simulink model "part2_sim5"  (R2019b)
settings: Solver=FixedStepAuto  StartTime=0.0  StopTime=1500  FixedStep=0.1  RelTol=1e-3
values from neighbouring files (symbols this model uses):
  Aw = [0 0 0 -0.487387871659 0 0 0 0 0 0 -0.487387871659 0 ... (36 elements, 6x6)]    [EKFData.mat]    (also in init_observer.m = [zeros(3,3) eye(3))
  C_w = [0 0 0 0 0 0 0 0 0 1 0 0 ... (18 elements, 3x6)]    [ExtendedKalmanFilter.mat]    (also in init_wind.m = C_w.data)
  counter = 1    [init_wind.m]    (also in plotVessel.m = 2; plotVessel_thrust.m = 2)
  Cw = [0 0 0 0 0 0 0 0 0 1 0 0 ... (18 elements, 3x6)]    [EKFData.mat]    (also in init_observer.m = [zeros(3,3) eye(3)])
  D = [264860  0  0; 0  881640  0; 0  0  337740000]    [EKFData.mat]    (also in ExtendedKalmanFilter.mat; init.m = [2.6486e5, 0, 0; 0, 8.8164e5 0; 0,0, 3.3774e8])
  eta_set = [0 50 50 0 0 0 0 -50 -50 0 0 0 ... (15 elements, 5x3)]    [EKFData.mat]    (also in ExtendedKalmanFilter.mat; init_autopilot.m = [0 0 0; 50 0 0;50 -50 0; 50 -50 -pi/4; 0 -50 -pi/4; 0 0 0]; main.m = [0 0 0; 0 0 0])
  gamma_m = [0.00394784176044  0  0; 0  0.00487387871659  0; 0  0  0.00394784176044]    [EKFData.mat]    (also in ExtendedKalmanFilter.mat; init_controller.m = [omega1^2 0 0; 0 omega2^2 0; 0 0 omega3^2])
  h_step = 0.1    [init_observer.m]
  K1 = [diag([k1,k2,k3]); diag([k4 k5 k6])]    [init_observer.m]
  K2 = diag([k7,k8,k9])    [init_observer.m]
  K3 = 0.1*K4    [init_observer.m]
  K4 = 0.01*diag([1 0.3 1]).*diag(M)    [init_observer.m]
  k_lqg = lqr(A_lqg,B_lqg,Q_lqg,P_lqg)    [init_controller.m]
  K_t = eye(8)    [init_thrustalloc.m]
  Kd_matrix = [4000000  0  0; 0  5000000  0; 0  0  80000]    [EKFData.mat]    (also in ExtendedKalmanFilter.mat; init_controller.m = [4*10^(6) 0 0 ; 0 5*10^(6) 0 ; 0 0 8*10^(4)])
  Ki_matrix = [200  0  0; 0  700  0; 0  0  1000]    [EKFData.mat]    (also in ExtendedKalmanFilter.mat; init_controller.m = [2*10^(2) 0 0 ; 0 7*10^(2) 0 ; 0 0 1*10^(3)])
  Kp_matrix = [200000  0  0; 0  400000  0; 0  0  10000000]    [EKFData.mat]    (also in ExtendedKalmanFilter.mat; init_controller.m = [2*10^(5) 0 0 ; 0 4*10^(5) 0 ; 0 0 1*10^(7)])
  M_inv = [1.46677031844e-07  0  0; 0  1.2695973473e-07  9.23036390732e-11; 0  9.23036390732e-11  2.80179152408e-10]    [EKFData.mat]    (also in ExtendedKalmanFilter.mat; init_observer.m = inv(M))
  mu = 0.001    [init_wind.m]
  noise_scalar = 1    [init_observer.m]
  omega_m = [0.125663706144  0  0; 0  0.125663706144  0; 0  0  0.125663706144]    [EKFData.mat]    (also in ExtendedKalmanFilter.mat; init_controller.m = [2*zeta1*omega1 0 0; 0 2*zeta2*omega2 0;0 0 2*zeta3*omega3])
  p = 1    [EKFData.mat]    (also in ExtendedKalmanFilter.mat; init_autopilot.m)
  P0 = [0 0 0 0 0 0 0 0 0 0 0 0 ... (225 elements, 15x15)]    [EKFData.mat]    (also in ExtendedKalmanFilter.mat = [10000000 0 0 0 0 0 0 0 0 0 0 0 ... (225 elements, 15x15)]; init_observer.m = diag(ones(1,15)))
  start_time = 0    [EKFData.mat]    (also in ExtendedKalmanFilter.mat; init_autopilot.m)
  t1 = 20    [EKFData.mat]    (also in ExtendedKalmanFilter.mat; init_controller.m)
  t2 = 10    [EKFData.mat]    (also in ExtendedKalmanFilter.mat; init_controller.m = 20)
  t3 = 20    [EKFData.mat]    (also in ExtendedKalmanFilter.mat; init_controller.m)
  Tb_1 = 1000    [EKFData.mat]    (also in ExtendedKalmanFilter.mat; init_observer.m)
  thrust_loc = [l_bt1, l_bt2, l_af, l_aa, b_s, b_p]    [init_thrustalloc.m]
  thrusters =     [EKFData.mat]    (also in ExtendedKalmanFilter.mat)
  time = 0    [EKFData.mat]    (also in ExtendedKalmanFilter.mat; init_autopilot.m; plotVessel.m = Eta.time(:); plotVessel_thrust.m = Sim2.data{eta_number}.Values.time)
  vessel =     [EKFData.mat]    (also in ExtendedKalmanFilter.mat)
  x0 = [0 0 0 0 0 0 0 0 0 1 1 1 ... (15 elements, 15x1)]    [EKFData.mat]    (also in ExtendedKalmanFilter.mat = [1 1 1 1 1 1 1 1 1 1 1 1 ... (15 elements, 15x1)]; init_observer.m = zeros(15,1))
undefined symbols (not defined in the file or in its folder): Hoerner, U_gust
libraries: marine_gnc x8, simulink x7, marine_hydro x2
settings Model: Creator=jonbjor  LastModifiedBy=yngve
settings DataIOCC: ReturnWorkspaceOutputs=off
settings DebuggingCC: ArithmeticOperatorsInVariantConditions=warning
settings SFSimCC: SimUseLocalCustomCode=off  CustomCodeUndefinedFunction=UseInterfaceOnly
settings RTWCC: RTWUseLocalCustomCode=off

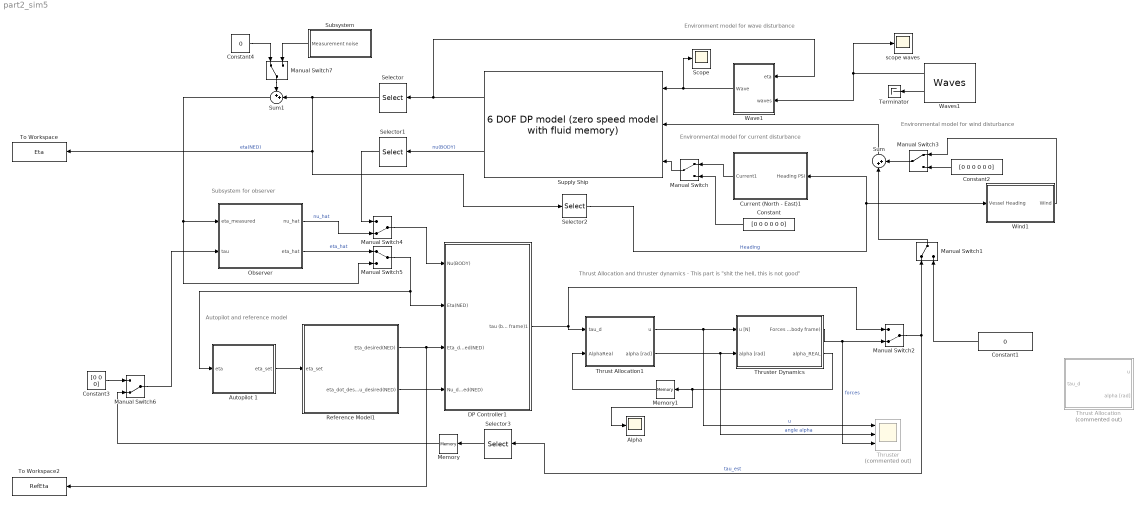
== system part2_sim5 ==
  note: Subsystem for observer
  note: Autopilot and reference model
  note: Environmental model for current disturbance
  note: Environmental model for wind disturbance
  note: Environment model for wave disturbance
  note: Thrust Allocation and thruster dynamics - This part is "shit the hell, this is not good"
  Alpha : Scope
  Autopilot 1 : Subsystem
  Constant : Constant  Value=[0 0 0 0 0 0]
  Constant1 : Constant  Value=0
  Constant2 : Constant  Value=[0 0 0 0 0 0]
  Constant3 : Constant  Value=[0 0 0]
  Constant4 : Constant  Value=0
  Current (North - East)1 : Subsystem
  DP Controller1 : Subsystem
  Manual Switch{,1,3,5,7} (5 alike) : ManualSwitch
  Manual Switch2 : ManualSwitch  CurrentSetting=0
  Manual Switch4 : ManualSwitch  CurrentSetting=0
  Manual Switch6 : ManualSwitch  CurrentSetting=0
  Memory : Memory  InheritSampleTime=on
  Memory1 : Memory  InitialCondition=[0 0 0 0 0]
  Observer : Subsystem
  Reference Model1 : Subsystem
  Scope : Scope
  Selector : Selector  InputPortWidth=6  IndexOptions=Index vector (dialog)  Indices=[1 2 6]  OutputSizes=1
  Selector1 : Selector  InputPortWidth=6  IndexOptions=Index vector (dialog)  Indices=[1 2 6]  OutputSizes=1
  Selector2 : Selector  InputPortWidth=3  IndexOptions=Index vector (dialog)  Indices=[3]  OutputSizes=1
  Selector3 : Selector  InputPortWidth=6  IndexOptions=Index vector (dialog)  Indices=[1 2 6]  OutputSizes=1
  Subsystem : Subsystem
  Sum : Sum  Inputs=|++
  Sum1 : Sum  Inputs=++|
  Supply Ship : marine_hydro/Hydro Library/6 DOF DP model  (zero speed model with fluid memory)  ABC=vesselABC  rho=1025  Axc=0.9*vessel.main.T*vessel.main.B  Ayc=0.9*vessel.main.T*vessel.main.Lpp  CX=1  CY_2D=Hoerner(vessel.main.B,vessel.main.T)  Bv=vessel.Bv  mask(6 DOF zero speed model){}
      link override "Integrator1 ": InitialCondition=nu0
      link override Integrator2: InitialCondition=eta0
      settings: SourceProductName=MSS Hydro
      mask Display:
      | image('supply.jpg');
      | color('white'); port_label('output', 1, 'eta')
      | color('white'); port_label('output', 2, 'nu')
      | color('white'); port_label('input', 1, 'tau_wave')
      | color('white'); port_label('input', 2, 'tau')
      | color('white'); port_label('input', 3, 'nu_c')
  Terminator : Terminator
  Thrust Allocation : Subsystem  Commented=on
  Thrust Allocation1 : Subsystem
  Thruster : Scope  Commented=on  NumInputPorts=3
  Thruster Dynamics : Subsystem  mask{thrusterfault=off}
      mask prompts: thrusterfault "Fault on thruster #2 and #5?"
  To Workspace : ToWorkspace  VariableName=Eta  SaveFormat=Timeseries  SampleTime=-1
  To Workspace2 : ToWorkspace  VariableName=RefEta  SaveFormat=Timeseries  SampleTime=-1
  Wave1 : Subsystem  mask{waveforces=on}
      mask prompts: waveforces "Waveforces enabled"
  Waves1 : marine_gnc/Environment/Waves/Waves  spectrum_type=Jonswap  disp_flag=on  plot_spectrum=off  plot_realization=off  hs=2.5  omega_peak=2*pi/9  psi_mean=225*pi/180  gamma=0  spread=2  depth=inf  nfreq=20  ndir=10  energylim=0.005  freq_cutoff=3  dir_cutoff=0  rand_seed=123  rand_freq=on  rand_dir=on  Zeta_a=0  Omega=0  Phase=0  Wavenum=0  Psi=0
      settings: SourceProductName=MSS GNC
  Wind1 : Subsystem
  "scope waves " : Scope
  wires:
  Selector/1 -> To Workspace/1, Selector2/1, Sum1/2  "eta(NED)"
  Observer/2(eta_hat) -> Manual Switch5/1  "eta_hat"
  Autopilot 1/1(eta_set) -> Reference Model1/1("eta_set ")
  Manual Switch1/1 -> Sum/1
  Constant/1 -> Manual Switch/2
  Manual Switch5/1 -> Autopilot 1/1(eta), DP Controller1/2("Eta(NED) ")
  Thruster Dynamics/1("Forces (body frame) ") -> Thruster/3, Manual Switch2/2  "forces"
  Supply Ship/1 -> Wave1/1(eta), Selector/1
  Manual Switch4/1 -> DP Controller1/1("Nu(BODY) ")
  Observer/1(nu_hat) -> Manual Switch4/2  "nu_hat"
  Manual Switch2/1 -> Selector3/1, Manual Switch1/1  "tau_est"
  Supply Ship/2 -> Selector1/1  "nu(BODY)"
  Selector1/1 -> Manual Switch4/1
  Constant2/1 -> Manual Switch3/2
  Manual Switch/1 -> Supply Ship/3
  Selector2/1 -> Current (North - East)1/1("Heading PSI "), Wind1/1(Vessel Heading)  "Heading"
  Manual Switch3/1 -> Sum/2
  Constant1/1 -> Manual Switch1/2
  Waves1/1 -> Wave1/2(waves), "scope waves "/1
  Wave1/1(Wave) -> Supply Ship/1, Scope/1
  Reference Model1/1(Eta_desired(NED)) -> DP Controller1/3("Eta_desired(NED) "), To Workspace2/1
  Thrust Allocation1/2(alpha [rad]) -> Thruster/2, Thruster Dynamics/2(alpha [rad])  "angle alpha"
  Thrust Allocation1/1(u) -> Thruster/1, Thruster Dynamics/1(u [N])  "u"
  Sum/1 -> Supply Ship/2
  Reference Model1/2(eta_dot_desired = nu_desired(NED)) -> DP Controller1/4(Nu_desired(NED))
  Wind1/1(Wind) -> Manual Switch3/1
  Current (North - East)1/1(Current1) -> Manual Switch/1
  Waves1/2 -> Terminator/1
  DP Controller1/1(tau (body frame)1) -> Thrust Allocation1/1(tau_d), Manual Switch2/1
  Manual Switch6/1 -> Observer/2(tau)
  Memory/1 -> Manual Switch6/2
  Constant3/1 -> Manual Switch6/1
  Sum1/1 -> Observer/1("eta_measured "), Manual Switch5/2
  Selector3/1 -> Memory/1
  Manual Switch7/1 -> Sum1/1
  Subsystem/1(Measurement noise) -> Manual Switch7/2
  Constant4/1 -> Manual Switch7/1
  Thruster Dynamics/2(alpha_REAL) -> Alpha/1, Memory1/1
  Memory1/1 -> Thrust Allocation1/2(AlphaReal)

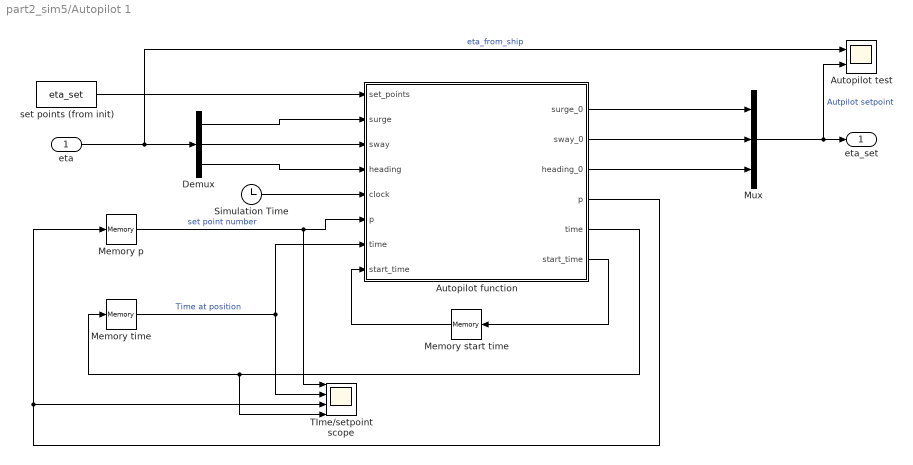
== system part2_sim5/Autopilot 1 ==
  eta : Inport
  "Autopilot function " : MATLAB Function  TreatAsAtomicUnit=on
  "Autopilot test " : Scope  NumInputPorts=2
  Demux : Demux  Outputs=3
  Memory start time : Memory  InitialCondition=start_time  InheritSampleTime=on
  Memory p : Memory  InitialCondition=p  InheritSampleTime=on
  Memory time : Memory  InitialCondition=time
  Mux : Mux  Inputs=3
  Simulation Time : Clock
  TIme/setpoint scope : Scope  NumInputPorts=4
  set points (from init) : Constant  Value=eta_set
  eta_set : Outport
  wires:
  set points (from init)/1 -> "Autopilot function "/1(set_points)
  Mux/1 -> "Autopilot test "/2, eta_set/1  "Autpilot setpoint"
  "Autopilot function "/1(surge_0) -> Mux/1
  eta/1 -> "Autopilot test "/1, Demux/1  "eta_from_ship"
  Demux/1 -> "Autopilot function "/2(surge)
  Demux/2 -> "Autopilot function "/3(sway)
  Simulation Time/1 -> "Autopilot function "/5(clock)
  Demux/3 -> "Autopilot function "/4(heading)
  "Autopilot function "/2(sway_0) -> Mux/2
  "Autopilot function "/3(heading_0) -> Mux/3
  Memory start time/1 -> "Autopilot function "/8("start_time ")
  "Autopilot function "/5(time) -> TIme/setpoint scope/4, Memory time/1
  Memory p/1 -> TIme/setpoint scope/1, "Autopilot function "/6("p ")  "set point number"
  "Autopilot function "/4(p) -> Memory p/1, TIme/setpoint scope/3
  Memory time/1 -> "Autopilot function "/7("time "), TIme/setpoint scope/2  "Time at position"
  "Autopilot function "/6(start_time) -> Memory start time/1

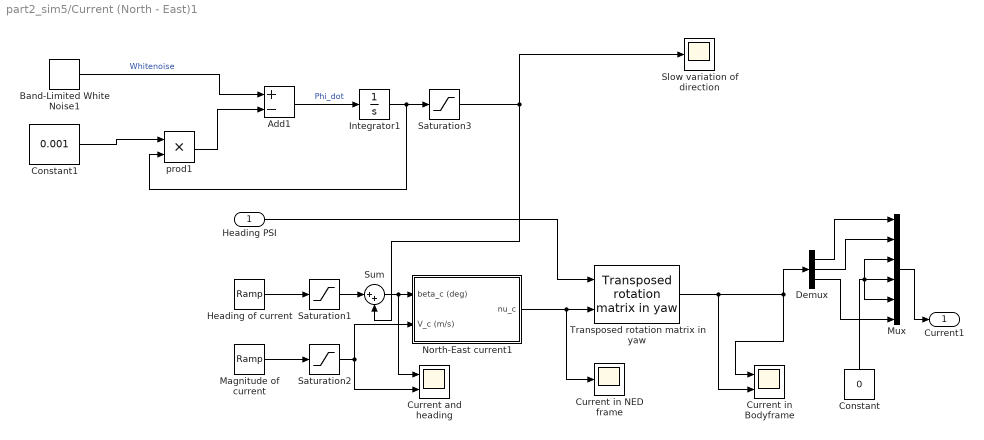
== system part2_sim5/Current (North - East)1 ==
  "Heading PSI " : Inport
  Add1 : Sum  Inputs=+-
  Band-Limited White Noise1 : simulink/Sources/Band-Limited White Noise  Cov=0.1  Ts=0.1  seed=[123456789]
  Constant : Constant  Value=0
  Constant1 : Constant  Value=0.001
  Current and heading : Scope  NumInputPorts=2
  "Current in Bodyframe " : Scope  NumInputPorts=2
  "Current in NED frame " : Scope
  Demux : Demux  Outputs=3
  "Heading of current " : simulink/Sources/Ramp  slope=0  start=0  InitialOutput=270
  Integrator1 : Integrator
  "Magnitude of current " : simulink/Sources/Ramp  slope=0  start=0  InitialOutput=0.2
  Mux : Mux  Inputs=6
  North-East current1 : Subsystem  AncestorBlock=marine_gnc/Environment/Current/North-East current
  Saturation1 : Saturate  UpperLimit=270  LowerLimit=180
  Saturation2 : Saturate  LowerLimit=0
  Saturation3 : Saturate  UpperLimit=5  LowerLimit=-5
  Slow variation of direction : Scope
  Sum : Sum  Inputs=|++
  Transposed rotation matrix in yaw : marine_gnc/Models/ Kinematics/Transposed rotation  matrix in yaw
      settings: SourceProductName=MSS GNC
  prod1 : Product  Inputs=**
  Current1 : Outport  VectorParamsAs1DForOutWhenUnconnected=off
  wires:
  Saturation2/1 -> North-East current1/2(V_c (m/s)), Current and heading/2
  "Magnitude of current "/1 -> Saturation2/1
  "Heading of current "/1 -> Saturation1/1
  Saturation1/1 -> Sum/1
  North-East current1/1(nu_c) -> Transposed rotation matrix in yaw/2, "Current in NED frame "/1
  Mux/1 -> Current1/1
  Constant/1 -> Mux/3, Mux/4, Mux/5
  Transposed rotation matrix in yaw/1 -> Demux/1, "Current in Bodyframe "/1, "Current in Bodyframe "/2
  "Heading PSI "/1 -> Transposed rotation matrix in yaw/1
  Add1/1 -> Integrator1/1  "Phi_dot"
  prod1/1 -> Add1/2
  Constant1/1 -> prod1/1
  Integrator1/1 -> Saturation3/1, prod1/2
  Band-Limited White Noise1/1 -> Add1/1  "Whitenoise"
  Saturation3/1 -> Sum/2, Slow variation of direction/1
  Sum/1 -> Current and heading/1, North-East current1/1(beta_c (deg))
  Demux/1 -> Mux/1
  Demux/2 -> Mux/2
  Demux/3 -> Mux/6

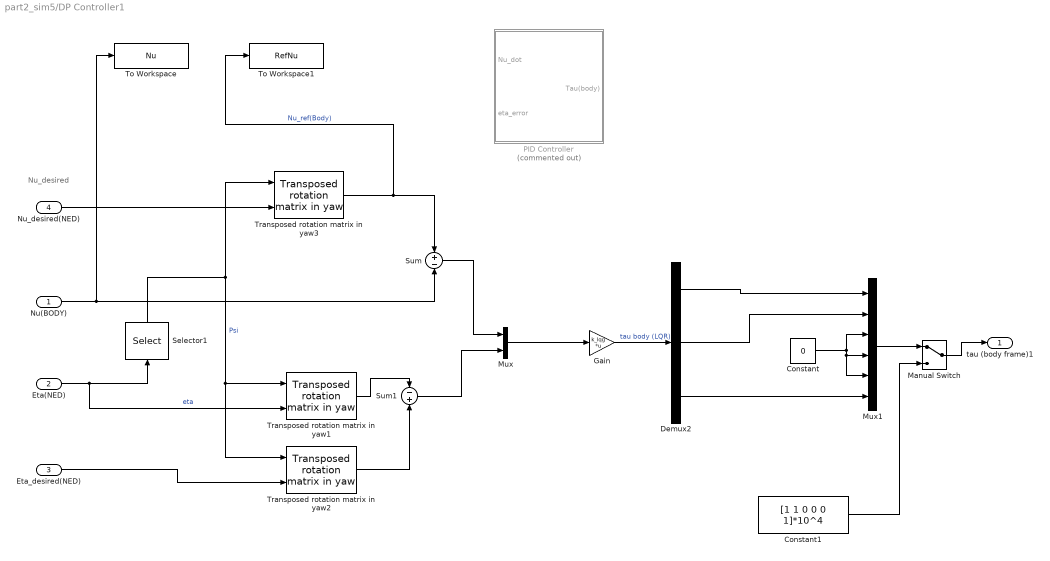
== system part2_sim5/DP Controller1 ==
  note: Nu_desired
  "Nu(BODY) " : Inport
  "Eta(NED) " : Inport  Port=2
  "Eta_desired(NED) " : Inport  Port=3
  Nu_desired(NED) : Inport  Port=4
  Constant : Constant  Value=0
  Constant1 : Constant  Value=[1 1 0 0 0 1]*10^4
  Demux2 : Demux  Outputs=3
  Gain : Gain  Gain=k_lqg  Multiplication=Matrix(K*u)
  Manual Switch : ManualSwitch
  Mux : Mux  Inputs=2
  Mux1 : Mux  Inputs=6
  "PID Controller " : Subsystem  Commented=on
  Selector1 : Selector  InputPortWidth=3  IndexOptions=Starting index (dialog)  Indices=[3]  OutputSizes=1
  Sum : Sum  Inputs=+-
  Sum1 : Sum  Inputs=-+
  To Workspace : ToWorkspace  VariableName=Nu  SaveFormat=Timeseries  SampleTime=-1
  To Workspace1 : ToWorkspace  VariableName=RefNu  SaveFormat=Timeseries  SampleTime=-1
  Transposed rotation matrix in yaw1 : marine_gnc/Models/ Kinematics/Transposed rotation  matrix in yaw
      settings: SourceProductName=MSS GNC
  Transposed rotation matrix in yaw2 : marine_gnc/Models/ Kinematics/Transposed rotation  matrix in yaw
      settings: SourceProductName=MSS GNC
  Transposed rotation matrix in yaw3 : marine_gnc/Models/ Kinematics/Transposed rotation  matrix in yaw
      settings: SourceProductName=MSS GNC
  tau (body frame)1 : Outport  VectorParamsAs1DForOutWhenUnconnected=off
  wires:
  Demux2/2 -> Mux1/2
  Selector1/1 -> Transposed rotation matrix in yaw3/1, Transposed rotation matrix in yaw2/1, Transposed rotation matrix in yaw1/1  "Psi"
  Constant/1 -> Mux1/5, Mux1/4, Mux1/3
  Demux2/1 -> Mux1/1
  "Eta(NED) "/1 -> Transposed rotation matrix in yaw1/2, Selector1/1  "eta"
  "Eta_desired(NED) "/1 -> Transposed rotation matrix in yaw2/2
  "Nu(BODY) "/1 -> To Workspace/1, Sum/2
  Nu_desired(NED)/1 -> Transposed rotation matrix in yaw3/2
  Demux2/3 -> Mux1/6
  Mux/1 -> Gain/1
  Sum/1 -> Mux/1
  Gain/1 -> Demux2/1  "tau body (LQR)"
  Transposed rotation matrix in yaw1/1 -> Sum1/1
  Sum1/1 -> Mux/2
  Transposed rotation matrix in yaw2/1 -> Sum1/2
  Transposed rotation matrix in yaw3/1 -> To Workspace1/1, Sum/1  "Nu_ref(Body)"
  Manual Switch/1 -> tau (body frame)1/1
  Mux1/1 -> Manual Switch/1
  Constant1/1 -> Manual Switch/2

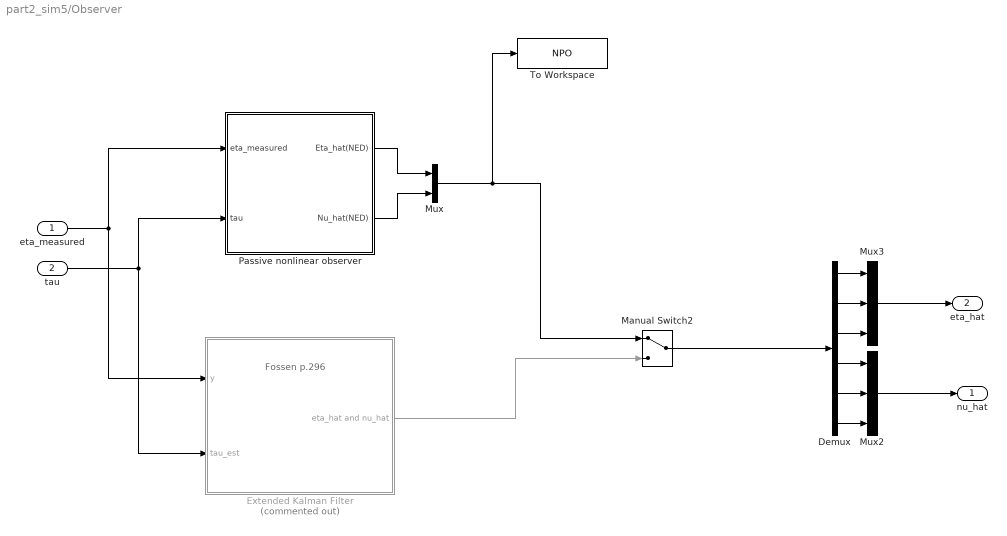
== system part2_sim5/Observer ==
  note: Fossen p.296
  "eta_measured " : Inport
  tau : Inport  Port=2  PortDimensions=[3 1]
  Demux : Demux  Outputs=6
  Extended Kalman Filter : Subsystem  Commented=on
      mask Display: image('Rudolf_Kalman.jpg'); % Use "Edit Image" on toolstrip to change.
  Manual Switch2 : ManualSwitch
  Mux : Mux  Inputs=2
  Mux2 : Mux  Inputs=3
  Mux3 : Mux  Inputs=3
  "Passive nonlinear observer " : Subsystem
  To Workspace : ToWorkspace  VariableName=NPO  SaveFormat=Timeseries  SampleTime=-1
  nu_hat : Outport
  eta_hat : Outport  Port=2
  wires:
  Extended Kalman Filter/1(eta_hat and nu_hat) -> Manual Switch2/2
  Demux/5 -> Mux2/2
  Manual Switch2/1 -> Demux/1
  Mux3/1 -> eta_hat/1
  Demux/1 -> Mux3/1
  Mux2/1 -> nu_hat/1
  Demux/3 -> Mux3/3
  Demux/6 -> Mux2/3
  Demux/4 -> Mux2/1
  Demux/2 -> Mux3/2
  tau/1 -> Extended Kalman Filter/2(tau_est), "Passive nonlinear observer "/2("tau ")
  "eta_measured "/1 -> Extended Kalman Filter/1(y), "Passive nonlinear observer "/1(eta_measured)
  "Passive nonlinear observer "/1("Eta_hat(NED) ") -> Mux/1
  "Passive nonlinear observer "/2("Nu_hat(NED) ") -> Mux/2
  Mux/1 -> To Workspace/1, Manual Switch2/1

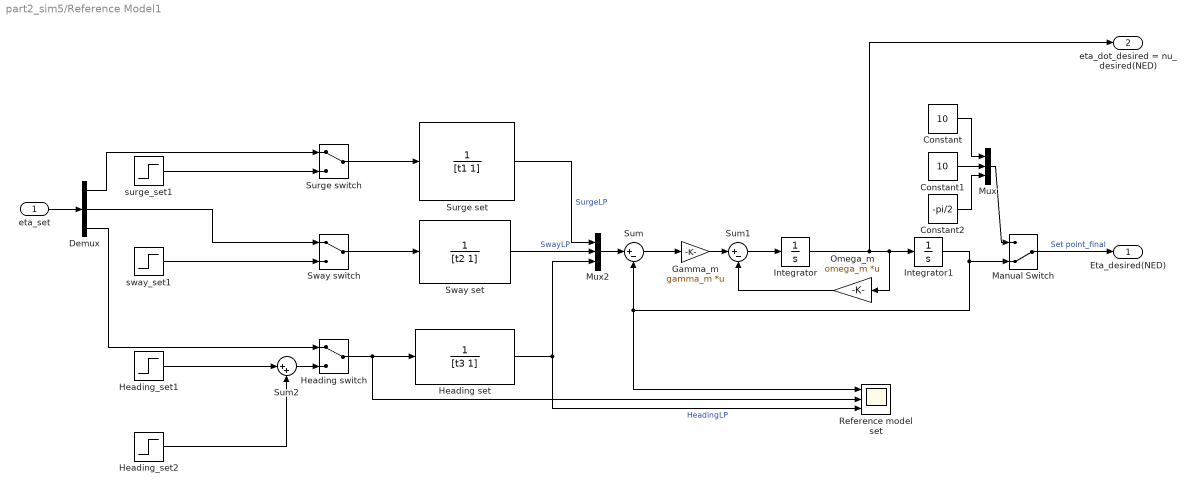
== system part2_sim5/Reference Model1 ==
  "eta_set " : Inport
  Constant : Constant  Value=10
  Constant1 : Constant  Value=10
  Constant2 : Constant  Value=-pi/2
  Demux : Demux  Outputs=3
  "Gamma_m " : Gain  Gain=gamma_m  Multiplication=Matrix(K*u)
  Heading set : TransferFcn  Denominator=[t3 1]
  "Heading switch " : ManualSwitch
  Heading_set1 : Step  Time=100  After=-pi/4  SampleTime=0
  Heading_set2 : Step  Time=800  After=pi/4  SampleTime=0
  Integrator : Integrator
  Integrator1 : Integrator
  Manual Switch : ManualSwitch  CurrentSetting=0
  Mux : Mux  Inputs=3
  Mux2 : Mux  Inputs=3
  Omega_m : Gain  Gain=omega_m  Multiplication=Matrix(K*u)
  "Reference model set " : Scope  NumInputPorts=3
  Sum : Sum  Inputs=|+-
  Sum1 : Sum  Inputs=|+-
  Sum2 : Sum  Inputs=|++
  Surge set : TransferFcn  Denominator=[t1 1]
  "Surge switch " : ManualSwitch
  Sway set : TransferFcn  Denominator=[t2 1]
  Sway switch : ManualSwitch
  "surge_set1 " : Step  Time=0  After=50  SampleTime=0
  sway_set1 : Step  Time=100  After=0  SampleTime=0
  Eta_desired(NED) : Outport  VectorParamsAs1DForOutWhenUnconnected=off
  eta_dot_desired = nu_desired(NED) : Outport  Port=2  VectorParamsAs1DForOutWhenUnconnected=off
  wires:
  Sum1/1 -> Integrator/1
  Surge set/1 -> Mux2/1  "SurgeLP"
  Sway set/1 -> Mux2/2  "SwayLP"
  Sum/1 -> "Gamma_m "/1
  Mux2/1 -> Sum/1
  Omega_m/1 -> Sum1/2
  Heading set/1 -> Mux2/3, "Reference model set "/3  "HeadingLP"
  "Gamma_m "/1 -> Sum1/1
  "Heading switch "/1 -> Heading set/1, "Reference model set "/2
  Integrator1/1 -> Manual Switch/2, "Reference model set "/1, Sum/2
  "eta_set "/1 -> Demux/1
  Demux/1 -> "Surge switch "/1
  "surge_set1 "/1 -> "Surge switch "/2
  "Surge switch "/1 -> Surge set/1
  Sway switch/1 -> Sway set/1
  sway_set1/1 -> Sway switch/2
  Demux/2 -> Sway switch/1
  Demux/3 -> "Heading switch "/1
  Heading_set1/1 -> Sum2/1
  Mux/1 -> Manual Switch/1
  Manual Switch/1 -> Eta_desired(NED)/1  "Set point_final"
  Constant/1 -> Mux/1
  Constant1/1 -> Mux/2
  Constant2/1 -> Mux/3
  Integrator/1 -> eta_dot_desired = nu_desired(NED)/1, Omega_m/1, Integrator1/1
  Sum2/1 -> "Heading switch "/2
  Heading_set2/1 -> Sum2/2

== system part2_sim5/Subsystem ==
  Band-Limited White Noise : simulink/Sources/Band-Limited White Noise  Cov=[0.01 0.01 0.01]  Ts=0.1  seed=[23341]
  Gain : Gain  Gain=noise_scalar
  Measurement noise : Outport
  wires:
  Band-Limited White Noise/1 -> Gain/1
  Gain/1 -> Measurement noise/1

== system part2_sim5/Thrust Allocation ==
  tau_d : Inport
  Constant : Constant  Value=K_t
  Constant1 : Constant  Value=thrust_loc
  MATLAB Function : MATLAB Function  TreatAsAtomicUnit=on
  Memory : Memory
  Selector : Selector  InputPortWidth=6  IndexOptions=Index vector (dialog)  Indices=[1 2 6]  OutputSizes=1
  u : Outport  VectorParamsAs1DForOutWhenUnconnected=off
  alpha [rad] : Outport  Port=2  VectorParamsAs1DForOutWhenUnconnected=off
  wires:
  tau_d/1 -> Selector/1
  MATLAB Function/1(u_thrust) -> u/1
  Constant/1 -> MATLAB Function/3(K_t)
  Constant1/1 -> MATLAB Function/2(thrust_loc)
  Selector/1 -> MATLAB Function/1(tau)
  MATLAB Function/2(alpha) -> alpha [rad]/1, Memory/1
  Memory/1 -> MATLAB Function/4(alpha_prev)

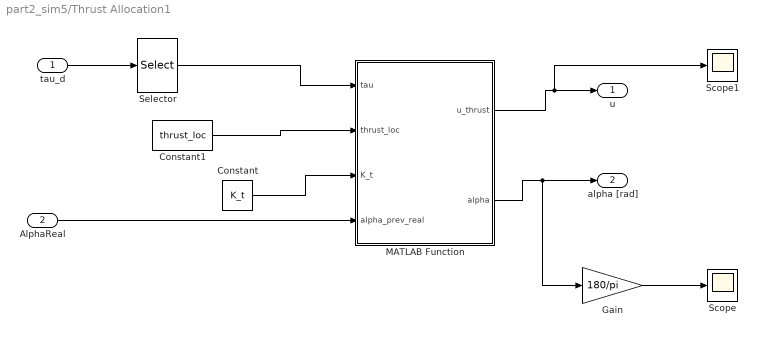
== system part2_sim5/Thrust Allocation1 ==
  tau_d : Inport
  AlphaReal : Inport  Port=2
  Constant : Constant  Value=K_t
  Constant1 : Constant  Value=thrust_loc
  Gain : Gain  Gain=180/pi
  MATLAB Function : MATLAB Function  TreatAsAtomicUnit=on
  Scope : Scope
  Scope1 : Scope
  Selector : Selector  InputPortWidth=6  IndexOptions=Index vector (dialog)  Indices=[1 2 6]  OutputSizes=1
  u : Outport  VectorParamsAs1DForOutWhenUnconnected=off
  alpha [rad] : Outport  Port=2  VectorParamsAs1DForOutWhenUnconnected=off
  wires:
  tau_d/1 -> Selector/1
  MATLAB Function/1(u_thrust) -> Scope1/1, u/1
  Selector/1 -> MATLAB Function/1(tau)
  MATLAB Function/2(alpha) -> Gain/1, alpha [rad]/1
  Gain/1 -> Scope/1
  Constant/1 -> MATLAB Function/3(K_t)
  Constant1/1 -> MATLAB Function/2(thrust_loc)
  AlphaReal/1 -> MATLAB Function/4(alpha_prev_real)

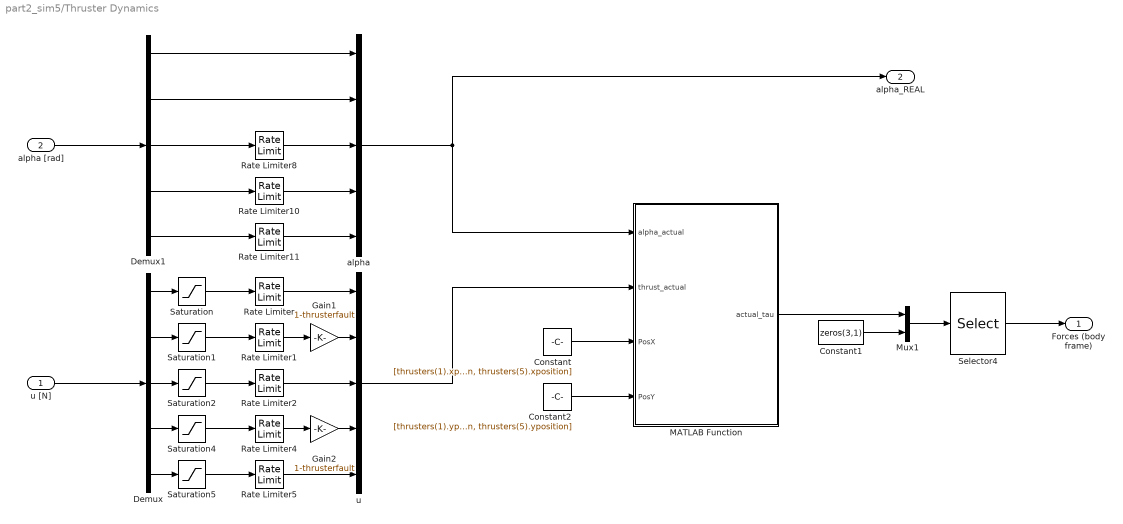
== system part2_sim5/Thruster Dynamics ==
  u [N] : Inport
  alpha [rad] : Inport  Port=2
  Constant : Constant  Value=[thrusters(1).xposition, thrusters(2).xposition, thrusters(3).xposition, thrusters(4).xposition, thrusters(5).xposition]
  Constant1 : Constant  Value=zeros(3,1)
  Constant2 : Constant  Value=[thrusters(1).yposition, thrusters(2).yposition, thrusters(3).yposition, thrusters(4).yposition, thrusters(5).yposition]
  Demux : Demux  Outputs=5
  Demux1 : Demux  Outputs=5
  Gain1 : Gain  Gain=1-thrusterfault
  Gain2 : Gain  Gain=1-thrusterfault
  MATLAB Function : MATLAB Function  TreatAsAtomicUnit=on
  Mux1 : Mux  Inputs=2
  Rate Limiter : RateLimiter  RisingSlewLimit=thrusters(1).rate  FallingSlewLimit=-thrusters(1).rate  SampleTimeMode=inherited
  Rate Limiter1 : RateLimiter  RisingSlewLimit=thrusters(2).rate  FallingSlewLimit=-thrusters(2).rate  SampleTimeMode=inherited
  Rate Limiter10 : RateLimiter  RisingSlewLimit=thrusters(4).rotationspeed  FallingSlewLimit=-thrusters(4).rotationspeed  SampleTimeMode=inherited
  Rate Limiter11 : RateLimiter  RisingSlewLimit=thrusters(5).rotationspeed  FallingSlewLimit=-thrusters(5).rotationspeed  SampleTimeMode=inherited
  Rate Limiter2 : RateLimiter  RisingSlewLimit=thrusters(3).rate  FallingSlewLimit=-thrusters(3).rate  SampleTimeMode=inherited
  Rate Limiter4 : RateLimiter  RisingSlewLimit=thrusters(4).rate  FallingSlewLimit=-thrusters(4).rate  SampleTimeMode=inherited
  Rate Limiter5 : RateLimiter  RisingSlewLimit=thrusters(5).rate  FallingSlewLimit=-thrusters(5).rate  SampleTimeMode=inherited
  Rate Limiter8 : RateLimiter  RisingSlewLimit=thrusters(3).rotationspeed  FallingSlewLimit=-thrusters(3).rotationspeed  SampleTimeMode=inherited
  Saturation : Saturate  UpperLimit=thrusters(1).thrust  LowerLimit=-thrusters(1).thrust
  Saturation1 : Saturate  UpperLimit=thrusters(2).thrust  LowerLimit=-thrusters(2).thrust
  Saturation2 : Saturate  UpperLimit=thrusters(3).thrust  LowerLimit=-thrusters(3).thrust
  Saturation4 : Saturate  UpperLimit=thrusters(4).thrust  LowerLimit=-thrusters(4).thrust
  Saturation5 : Saturate  UpperLimit=thrusters(5).thrust  LowerLimit=-thrusters(5).thrust
  Selector4 : Selector  InputPortWidth=6  IndexOptions=Index vector (dialog)  Indices=[1 2 4 5 6 3]  OutputSizes=1
  alpha : Mux  Inputs=5
  u : Mux  Inputs=5
  "Forces (body frame) " : Outport  VectorParamsAs1DForOutWhenUnconnected=off
  alpha_REAL : Outport  Port=2  VectorParamsAs1DForOutWhenUnconnected=off
  wires:
  Rate Limiter2/1 -> u/3
  Saturation/1 -> Rate Limiter/1
  Mux1/1 -> Selector4/1
  Constant1/1 -> Mux1/2
  Saturation4/1 -> Rate Limiter4/1
  Demux/2 -> Saturation1/1
  Saturation1/1 -> Rate Limiter1/1
  Demux/1 -> Saturation/1
  Demux/3 -> Saturation2/1
  Saturation2/1 -> Rate Limiter2/1
  Selector4/1 -> "Forces (body frame) "/1
  Gain1/1 -> u/2
  Rate Limiter1/1 -> Gain1/1
  Rate Limiter/1 -> u/1
  Rate Limiter4/1 -> Gain2/1
  Saturation5/1 -> Rate Limiter5/1
  Rate Limiter8/1 -> alpha/3
  u [N]/1 -> Demux/1
  alpha [rad]/1 -> Demux1/1
  Constant/1 -> MATLAB Function/3(PosX)
  Constant2/1 -> MATLAB Function/4(PosY)
  u/1 -> MATLAB Function/2(thrust_actual)
  alpha/1 -> MATLAB Function/1(alpha_actual), alpha_REAL/1
  MATLAB Function/1(actual_tau) -> Mux1/1
  Demux1/3 -> Rate Limiter8/1
  Rate Limiter10/1 -> alpha/4
  Demux1/4 -> Rate Limiter10/1
  Demux1/5 -> Rate Limiter11/1
  Rate Limiter11/1 -> alpha/5
  Demux1/2 -> alpha/2
  Demux1/1 -> alpha/1
  Gain2/1 -> u/4
  Demux/4 -> Saturation4/1
  Demux/5 -> Saturation5/1
  Rate Limiter5/1 -> u/5

== system part2_sim5/Wave1 ==
  eta : Inport
  waves : Inport  Port=2
  Gain : Gain  Gain=waveforces
  Sum : Sum
  Wave loads (U=0) : marine_hydro/Hydro Library/Wave loads (U=0)  SystemSampleTime=-1  Latency=0  AutoFrameSizeCalculation=off
      settings: SourceProductName=MSS Hydro
  Wave : Outport  VectorParamsAs1DForOutWhenUnconnected=off
  wires:
  eta/1 -> Wave loads (U=0)/1
  waves/1 -> Wave loads (U=0)/2
  Sum/1 -> Gain/1
  Wave loads (U=0)/1 -> Sum/1
  Wave loads (U=0)/2 -> Sum/2
  Gain/1 -> Wave/1

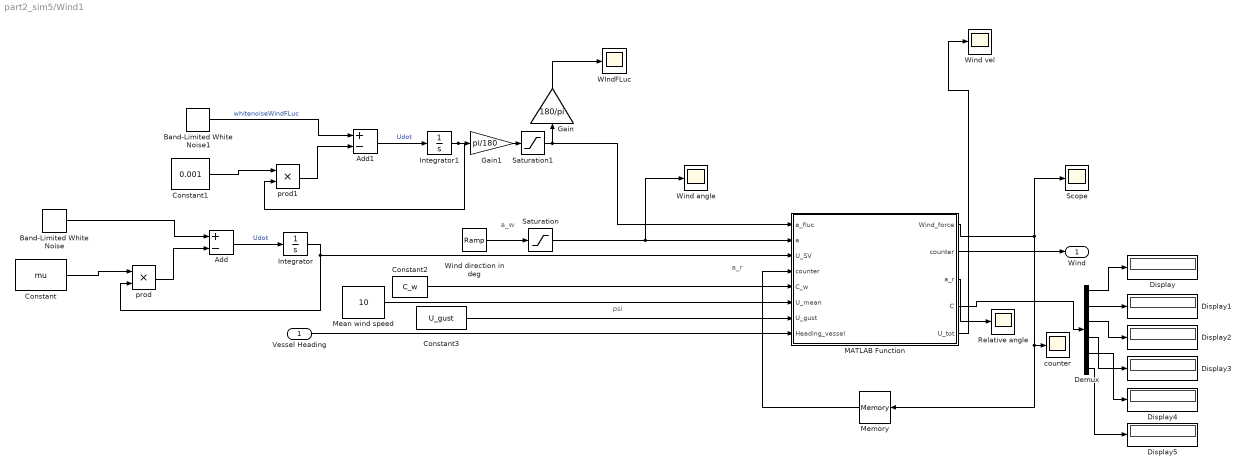
== system part2_sim5/Wind1 ==
  note: a_r
  note: psi
  note: a_w
  Vessel Heading : Inport
  Add : Sum  Inputs=+-
  Add1 : Sum  Inputs=+-
  Band-Limited White Noise : simulink/Sources/Band-Limited White Noise  Cov=w  Ts=0.1  seed=[23341]
  Band-Limited White Noise1 : simulink/Sources/Band-Limited White Noise  Cov=0.1  Ts=0.1  seed=[123456789]
  Constant : Constant  Value=mu
  Constant1 : Constant  Value=0.001
  Constant2 : Constant  Value=C_w
  Constant3 : Constant  Value=U_gust
  Demux : Demux  Outputs=6
  Display{,1..5} (6 alike) : Display
  Gain : Gain  Gain=180/pi
  Gain1 : Gain  Gain=pi/180
  Integrator : Integrator
  Integrator1 : Integrator
  MATLAB Function : MATLAB Function  TreatAsAtomicUnit=on
  Mean wind speed : Constant  Value=10
  Memory : Memory  InitialCondition=counter  InheritSampleTime=on
  "Relative angle " : Scope
  Saturation : Saturate  UpperLimit=2*pi  LowerLimit=0
  Saturation1 : Saturate  UpperLimit=5*pi/180  LowerLimit=-5*pi/180
  Scope : Scope
  "WIndFLuc " : Scope
  Wind angle : Scope
  Wind direction in deg : simulink/Sources/Ramp  slope=0  start=0  InitialOutput=pi
  "Wind vel " : Scope
  counter : Scope
  prod : Product  Inputs=**
  prod1 : Product  Inputs=**
  Wind : Outport  VectorParamsAs1DForOutWhenUnconnected=off
  wires:
  Vessel Heading/1 -> MATLAB Function/8(Heading_vessel)
  Saturation/1 -> Wind angle/1, MATLAB Function/2(a)
  Wind direction in deg/1 -> Saturation/1
  Add/1 -> Integrator/1  "Udot"
  Constant/1 -> prod/1
  Integrator/1 -> prod/2, MATLAB Function/3(U_SV)
  Band-Limited White Noise/1 -> Add/1
  prod/1 -> Add/2
  Memory/1 -> MATLAB Function/4("counter ")
  MATLAB Function/2(counter) -> Memory/1, counter/1
  Constant1/1 -> prod1/1
  Band-Limited White Noise1/1 -> Add1/1  "whitenoiseWindFLuc"
  prod1/1 -> Add1/2
  Integrator1/1 -> prod1/2, Gain1/1
  Add1/1 -> Integrator1/1  "Udot"
  MATLAB Function/1(Wind_force) -> Wind/1, Scope/1
  Constant2/1 -> MATLAB Function/5(C_w)
  Mean wind speed/1 -> MATLAB Function/6(U_mean)
  Constant3/1 -> MATLAB Function/7(U_gust)
  MATLAB Function/3(a_r) -> "Relative angle "/1
  Demux/1 -> Display/1
  Demux/2 -> Display1/1
  Demux/3 -> Display2/1
  Demux/4 -> Display3/1
  Demux/5 -> Display4/1
  Demux/6 -> Display5/1
  MATLAB Function/4(C) -> Demux/1
  MATLAB Function/5(U_tot) -> "Wind vel "/1
  Gain/1 -> "WIndFLuc "/1
  Saturation1/1 -> MATLAB Function/1(a_fluc), Gain/1
  Gain1/1 -> Saturation1/1

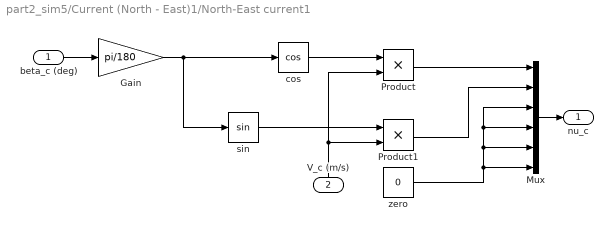
== system part2_sim5/Current (North - East)1/North-East current1 ==
  beta_c (deg) : Inport
  V_c (m/s) : Inport  Port=2
  Gain : Gain  Gain=pi/180
  Mux : Mux  Inputs=6
  Product : Product  RndMeth=Zero
  Product1 : Product  RndMeth=Zero
  cos : Trigonometry  Operator=cos
  sin : Trigonometry
  zero : Constant  Value=0
  nu_c : Outport
  wires:
  Mux/1 -> nu_c/1
  beta_c (deg)/1 -> Gain/1
  zero/1 -> Mux/6, Mux/5, Mux/4, Mux/3
  Product1/1 -> Mux/2
  Product/1 -> Mux/1
  sin/1 -> Product1/1
  V_c (m/s)/1 -> Product1/2, Product/2
  cos/1 -> Product/1
  Gain/1 -> cos/1, sin/1

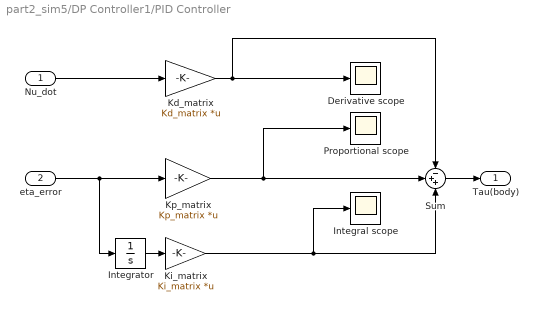
== system part2_sim5/DP Controller1/PID Controller  ==
  "Nu_dot " : Inport
  "eta_error " : Inport  Port=2
  "Derivative scope " : Scope
  "Integral scope " : Scope
  Integrator : Integrator
  "Kd_matrix " : Gain  Gain=Kd_matrix  Multiplication=Matrix(K*u)
  "Ki_matrix " : Gain  Gain=Ki_matrix  Multiplication=Matrix(K*u)
  Kp_matrix : Gain  Gain=Kp_matrix  Multiplication=Matrix(K*u)
  "Proportional scope " : Scope
  Sum : Sum  Inputs=-++
  Tau(body) : Outport  VectorParamsAs1DForOutWhenUnconnected=off
  wires:
  "eta_error "/1 -> Integrator/1, Kp_matrix/1
  "Nu_dot "/1 -> "Kd_matrix "/1
  Integrator/1 -> "Ki_matrix "/1
  Kp_matrix/1 -> "Proportional scope "/1, Sum/2
  "Kd_matrix "/1 -> Sum/1, "Derivative scope "/1
  Sum/1 -> Tau(body)/1
  "Ki_matrix "/1 -> Sum/3, "Integral scope "/1

== system part2_sim5/Observer/Extended Kalman Filter ==
  y : Inport
  tau_est : Inport  Port=2
  Extended Kalman Filter : MATLAB Function  TreatAsAtomicUnit=on  SystemSampleTime=h_step
  Memory : Memory  InitialCondition=x0
  Memory1 : Memory  InitialCondition=P0
  Selector : Selector  InputPortWidth=15  IndexOptions=Index vector (dialog)  Indices=[7 8 9 13 14 15]  OutputSizes=1
  Terminator : Terminator  Commented=on
  eta_hat and nu_hat : Outport
  wires:
  Extended Kalman Filter/4(x_bar) -> Memory/1
  Extended Kalman Filter/3(P_bar) -> Memory1/1
  Memory1/1 -> Extended Kalman Filter/3("P_bar ")
  Memory/1 -> Extended Kalman Filter/4("x_bar ")
  Extended Kalman Filter/2(x_hat) -> Selector/1
  y/1 -> Extended Kalman Filter/1(y)
  Selector/1 -> eta_hat and nu_hat/1
  Extended Kalman Filter/1(P_hat) -> Terminator/1
  tau_est/1 -> Extended Kalman Filter/2(tau)

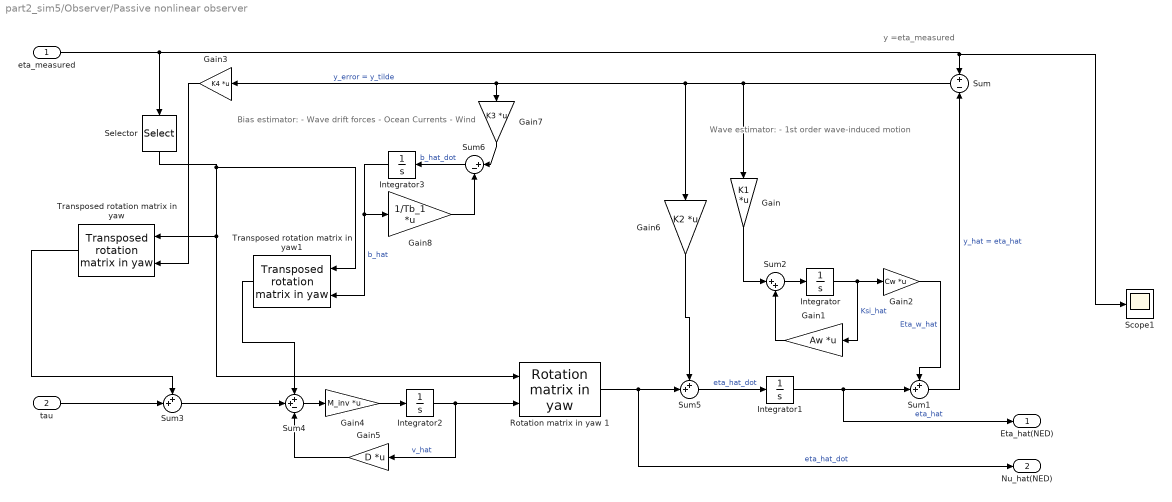
== system part2_sim5/Observer/Passive nonlinear observer  ==
  note: y =eta_measured
  note: Wave estimator:
      | - 1st order wave-induced motion
  note: Bias estimator:
      | - Wave drift forces
      | - Ocean Currents
      | - Wind
  eta_measured : Inport
  "tau " : Inport  Port=2
  Gain : Gain  Gain=K1  Multiplication=Matrix(K*u)
  Gain1 : Gain  Gain=Aw  Multiplication=Matrix(K*u)
  Gain2 : Gain  Gain=Cw  Multiplication=Matrix(K*u)
  Gain3 : Gain  Gain=K4  Multiplication=Matrix(K*u)
  Gain4 : Gain  Gain=M_inv  Multiplication=Matrix(K*u)
  Gain5 : Gain  Gain=D  Multiplication=Matrix(K*u)
  Gain6 : Gain  Gain=K2  Multiplication=Matrix(K*u)
  Gain7 : Gain  Gain=K3  Multiplication=Matrix(K*u)
  Gain8 : Gain  Gain=1/Tb_1  Multiplication=Matrix(K*u)
  Integrator{,1..3} (4 alike) : Integrator
  Rotation matrix in yaw 1 : marine_gnc/Models/ Kinematics/Rotation matrix in yaw 
      settings: SourceProductName=MSS GNC
  Scope1 : Scope
  Selector : Selector  InputPortWidth=3  IndexOptions=Index vector (dialog)  Indices=[3]  OutputSizes=1
  Sum : Sum  Inputs=+-
  Sum1 : Sum  Inputs=++|
  Sum2 : Sum  Inputs=|++
  Sum3 : Sum  Inputs=++|
  Sum4 : Sum  Inputs=++-
  Sum5 : Sum  Inputs=++|
  Sum6 : Sum  Inputs=|+-
  Transposed rotation matrix in yaw : marine_gnc/Models/ Kinematics/Transposed rotation  matrix in yaw
      settings: SourceProductName=MSS GNC
  Transposed rotation matrix in yaw1 : marine_gnc/Models/ Kinematics/Transposed rotation  matrix in yaw
      settings: SourceProductName=MSS GNC
  "Eta_hat(NED) " : Outport
  "Nu_hat(NED) " : Outport  Port=2
  wires:
  eta_measured/1 -> Selector/1, Scope1/1, Sum/1
  Gain/1 -> Sum2/1
  Sum2/1 -> Integrator/1
  Integrator/1 -> Gain2/1, Gain1/1  "Ksi_hat"
  Gain1/1 -> Sum2/2
  Gain2/1 -> Sum1/1  "Eta_w_hat"
  "tau "/1 -> Sum3/2
  Transposed rotation matrix in yaw/1 -> Sum3/1
  Sum3/1 -> Sum4/2
  Transposed rotation matrix in yaw1/1 -> Sum4/1
  Sum4/1 -> Gain4/1
  Gain4/1 -> Integrator2/1
  Integrator2/1 -> Rotation matrix in yaw 1/2, Gain5/1  "v_hat"
  Gain5/1 -> Sum4/3
  Rotation matrix in yaw 1/1 -> "Nu_hat(NED) "/1, Sum5/2  "eta_hat_dot"
  Sum5/1 -> Integrator1/1  "eta_hat_dot"
  Gain6/1 -> Sum5/1
  Sum/1 -> Gain/1, Gain6/1, Gain3/1, Gain7/1  "y_error = y_tilde"
  Gain7/1 -> Sum6/1
  Gain8/1 -> Sum6/2
  Selector/1 -> Transposed rotation matrix in yaw/1, Rotation matrix in yaw 1/1, Transposed rotation matrix in yaw1/1
  Integrator3/1 -> Gain8/1, Transposed rotation matrix in yaw1/2  "b_hat"
  Gain3/1 -> Transposed rotation matrix in yaw/2
  Sum1/1 -> Sum/2  "y_hat = eta_hat"
  Integrator1/1 -> Sum1/2, "Eta_hat(NED) "/1  "eta_hat"
  Sum6/1 -> Integrator3/1  "b_hat_dot"

== matlab function part2_sim5/Thrust Allocation/MATLAB Function ==
  data: tau input; thrust_loc input; K_t input; u_thrust output; alpha output; alpha_prev input
function [u_thrust, alpha] = thrust_allocation_extended(tau, thrust_loc, K_t, alpha_prev)
%Calculates the control vector for each thruster
%thrust_loc = [l_bt1, l_bt2, l_af, l_aa, b_s, b_p]; 

T_extended = [0 0 1 0 1 0 1 0; ...
    1 1 0 1 0 1 0 1; 
    thrust_loc(1) thrust_loc(2) 0 thrust_loc(3) thrust_loc(5) ...
    thrust_loc(4) thrust_loc(6) thrust_loc(4)]; 


u_e = inv(K_t)*pinv(T_extended)*tau;

u_d_3 = sqrt(u_e(3)^2 + u_e(4)^2); %Azimuth forward
u_d_4 = sqrt(u_e(5)^2 + u_e(6)^2); %Azimuth stern, starboard
u_d_5 = sqrt(u_e(7)^2 + u_e(8)^2); %Azimuth stern, port


%Thrust angles, alpha
alpha = zeros(5, 1); 
alpha(1) = pi/2;                     %Tunnel thruster 1
alpha(2) = pi/2;                     %Tunnel thruster 2
alpha(3) = atan2(u_e(4), u_e(3));    %Azimuth forward
alpha(4) = atan2(u_e(6), u_e(5));    %Azimuth aft, starboard
alpha(5) = atan2(u_e(8), u_e(7));    %Azimuth aft, port

u_extended = [u_e(1); u_e(2); u_d_3; u_d_4; u_d_5];
    
%Singular value handling
% T_alpha = [0 0 cos(alpha(3)) cos(alpha(4)) cos(alpha(5)); ...
%     1 1 sin(alpha(3)) sin(alpha(4)) sin(alpha(5)); ...
%     thrust_loc(1) thrust_loc(2) thrust_loc(3) ...
%     -thrust_loc(4)*sin(alpha(4))-thrust_loc(5)*cos(alpha(4))...
%     -thrust_loc(4)*sin(alpha(5))-thrust_loc(6)*cos(alpha(5))]; 
% 
% u_alpha = pinv(T_alpha)*tau; 

u_thrust = u_extended;

for i = 1:5 
    if (alpha_prev(i) <= -pi)
        alpha_prev(i) = 2*pi+alpha_prev(i); 
    elseif (alpha_prev(i) >= pi)
        alpha_prev(i) = -(2*pi - alpha_prev(i));
    end
end

rot_speed = 0.1*pi/30;  %2 rpm & 0.1 sec run time  

if (alpha(3) > alpha_prev(3) + rot_speed)
    alpha(3) = alpha_prev(3) + rot_speed; 
elseif (alpha(3) < alpha_prev(3) - rot_speed)
    alpha(3) = alpha_prev(3)-rot_speed; 
end
if (alpha(4) > alpha_prev(4) + rot_speed)
    alpha(4) = alpha_prev(4) + rot_speed; 
elseif (alpha(4) < alpha_prev(4) - rot_speed)
    alpha(4) = alpha_prev(4)-rot_speed; 
end
if (alpha(5) > alpha_prev(5) + rot_speed)
    alpha(5) = alpha_prev(5) + rot_speed; 
elseif (alpha(5) < alpha_prev(5) - rot_speed)
    alpha(5) = alpha_prev(5)-rot_speed; 
end

%Checking forbidden sectors: 
    %Azimuth aft, starboard
    if alpha(4, 1) > pi/4 && alpha(4, 1) <= 3*pi/8 %Upper half of sector
        alpha(4, 1) = pi/4; 
    elseif alpha(4, 1) > 3*pi/8 && alpha(4, 1) < pi/2 %Lower half of sector
        alpha(4, 1) = pi/2; 
    end
    if alpha(5, 1) > -pi/4 && alpha(5, 1) <= -3*pi/8 %Upper half of sector
        alpha(5, 1) = -pi/4; 
    elseif alpha(5, 1) > -3*pi/8 && alpha(5, 1) < -pi/2 %Lower half of sector
        alpha(5, 1) = -pi/2; 
    end

end

== matlab function part2_sim5/Thrust Allocation1/MATLAB Function ==
  data: tau input; u_thrust output; alpha output; thrust_loc input; K_t input; alpha_prev_real input
function [u_thrust, alpha] = thrust_allocation_extended(tau, thrust_loc, K_t, alpha_prev_real)
%Calculates the control vector for each thruster

T_extended = [0 0 1 0 1 0 1 0; ...
    1 1 0 1 0 1 0 1; 
    thrust_loc(1) thrust_loc(2) 0 thrust_loc(3) thrust_loc(5) thrust_loc(4) thrust_loc(6) thrust_loc(4)]; 

u_e = inv(K_t)*pinv(T_extended)*tau;

u_d_3 = sqrt(u_e(3)^2 + u_e(4)^2); %Azimuth forward
u_d_4 = sqrt(u_e(5)^2 + u_e(6)^2); %Azimuth stern, starboard
u_d_5 = sqrt(u_e(7)^2 + u_e(8)^2); %Azimuth stern, port

%Thrust angles, alpha
alpha = zeros(5, 1); 
alpha(1) = pi/2;                     %Tunnel thruster 1
alpha(2) = pi/2;                     %Tunnel thruster 2
alpha(3) = atan2(u_e(4), u_e(3));    %Azimuth forward
alpha(4) = atan2(u_e(6), u_e(5));    %Azimuth aft, starboard
alpha(5) = atan2(u_e(8), u_e(7));    %Azimuth aft, port

u_thrust = [u_e(1); u_e(2); u_d_3; u_d_4; u_d_5];

%Limiting thrust to azimuths under heavy position change
for i = 3:5
   
%    if(i == 4 &&  (alpha(i, 1) > pi/3 && alpha(i, 1) <= pi/2) || (alpha(i, 1) > pi/2 && alpha(i, 1) < 2*pi/3))
%        
%    elseif(i==5 &&    (alpha(5, 1) >= -pi/2 && alpha(5, 1) < -pi/3) || (alpha(5, 1) > -2*pi/3 && alpha(5, 1) < -pi/2))
   %elseif    
   if(alpha(i) > alpha_prev_real(i) + 10*pi/180 || alpha(i) < alpha_prev_real(i) - 10*pi/180)
      u_thrust(i) = 0; 
       
   end
end

%Checking forbidden sectors: 
    %Azimuth stern, starboard
    if alpha(4, 1) > pi/3 && alpha(4, 1) <= pi/2 %Upper half of sector
        alpha(4, 1) = pi/3; 

    elseif alpha(4, 1) > pi/2 && alpha(4, 1) < 2*pi/3 %Lower half of sector
        alpha(4, 1) = 2*pi/3; 
    end
    %Azimuth stern, port
    if alpha(5, 1) >= -pi/2 && alpha(5, 1) < -pi/3 %Upper half of sector
        alpha(5, 1) = -pi/3; 
    elseif alpha(5, 1) > -2*pi/3 && alpha(5, 1) < -pi/2 %Lower half of sector
        alpha(5, 1) = -2*pi/3; 
    end
    
            
% T_alpha = [0 0 cos(alpha(3)) cos(alpha(4)) cos(alpha(5)); ...
%     1 1 sin(alpha(3)) sin(alpha(4)) sin(alpha(5)); ...
%     thrust_loc(1) thrust_loc(2) thrust_loc(3) ...
%     -thrust_loc(4)*sin(alpha(4))-thrust_loc(5)*cos(alpha(4))...
%     -thrust_loc(4)*sin(alpha(5))-thrust_loc(6)*cos(alpha(5))]; 
% K_alpha = eye(5);
% 
% u_alpha = inv(K_alpha)*pinv(T_alpha)*tau; 
% 
% u_thrust = u_alpha;
end

== matlab function part2_sim5/Wind1/MATLAB Function ==
  data: a_fluc input; a input; Wind_force output; U_SV input; counter input; counter output; C_w input; U_mean input; U_gust input; a_r output; Heading_vessel input; C output; U_tot output
function [Wind_force,counter, a_r,C,U_tot]  = fcn(a_fluc, a,U_SV,counter, C_w, U_mean, U_gust,Heading_vessel)
counter = counter + 1;
a_r = 0; %relative angle
Wind_force = [0 0 0 0 0 0]';

C_x = 0;
C_y = 0;
C_z = 0;
C_theta = 0;
C_phi= 0;
C_psi = 0;
C = zeros(6,1);

%Se om vinkelen er mellom 0 og 2pi
a_r = a+a_fluc-Heading_vessel;
%For testing purpose:
%a_r = u;

%Så hente ut tilhørende verdier fra appendix A
temp = a_r*180/pi;
for i = 1:(length(C_w)-1)
    if(temp >=C_w(i,1)  &&temp <C_w(i+1,1))
C_x = C_w(i,2);
C_y = C_w(i,3);
C_z = C_w(i,4);
C_theta = C_w(i,5);
C_phi= C_w(i,6);
C_psi = C_w(i,7);


    end


%Total wind velocity
U_tot = U_mean + U_SV + U_gust(counter);
    %coefficient matrix
C = [C_x,C_y,C_z,C_theta,C_phi,C_psi]';

Wind_force = abs(U_tot)^2*[C(1),C(2),C(3),C(4),C(5),C(6)]';


end

== matlab function part2_sim5/Thruster Dynamics/MATLAB Function ==
  data: alpha_actual input; thrust_actual input; actual_tau output; PosX input; PosY input
function actual_tau   = fcn(alpha_actual,thrust_actual,PosX,PosY)

    Alpha_surge =[cos(alpha_actual(1)) cos(alpha_actual(2)) cos(alpha_actual(3)) cos(alpha_actual(4)) cos(alpha_actual(5))];  
    Alpha_sway = [sin(alpha_actual(1)) sin(alpha_actual(2)) sin(alpha_actual(3)) sin(alpha_actual(4)) sin(alpha_actual(5))];
    Alpha_yaw = [sin(alpha_actual(1))*PosX(1)-cos(alpha_actual(1))*PosY(1) sin(alpha_actual(2))*PosX(2)-cos(alpha_actual(2))*PosY(2) ...
                 sin(alpha_actual(3))*PosX(3)-cos(alpha_actual(3))*PosY(3) sin(alpha_actual(4))*PosX(4)-cos(alpha_actual(4))*PosY(4) ...
                 sin(alpha_actual(5))*PosX(5)-cos(alpha_actual(5))*PosY(5)];

    actual_tau = [Alpha_surge; Alpha_sway; Alpha_yaw]*thrust_actual;
end

== matlab function part2_sim5/Autopilot 1/Autopilot function  ==
  data: set_points input; surge_0 output; surge input; sway input; heading input; clock input; sway_0 output; heading_0 output; p input; time input; start_time input; p output; time output; start_time output
function [surge_0, sway_0, heading_0, p, time, start_time] = autopilot(set_points, surge, sway, heading, clock, p, time, start_time)
%Inputs current surge, sway, heading and outputs ref values surge_0,
%sway_0, heading_0

time_crit = 30;  %Time criteria at set point before moving
accu = 5;       %Accuracy/Tollerance
accu_h = 5 * pi/180;   %Heading accuracy



dim = size(set_points);

if p >= dim(1)
    time = 0; 
else
    %Checking positions: 
    if (set_points(p, 1)-accu) <= surge && surge <= (set_points(p, 1) + accu)

        if (set_points(p, 3)-accu_h) <= heading && heading...
                <= (set_points(p, 3)+ accu_h)

            if (set_points(p, 2)-accu) <= sway && sway...
                    <= (set_points(p, 2)+ accu)
%Checking if vessel is at desired position for desired amount of time
                if time == 0
                   start_time = clock;  %Start time of counting time in pos.
                   time = 0.1; %simulation step time
                else%Counting time at position
                    time = (clock-start_time);     %Counting time at position
                end
                if time >= time_crit
                    p = p + 1;    %Incrementing the set point 
                    if p > dim(1)
                        p = dim(1);     %Last point met
                    end
                    time = 0;                   %Zeroing time counter
                end
            else
                time = 0;   %No longer in correct position, stop counting. 
            end
        else
            time = 0; 
        end
    else
        time = 0; 
    end
end

%Setting referance points: 
surge_0 = set_points(p, 1); 
sway_0 = set_points(p, 2); 
heading_0 = set_points(p, 3);  

end

== matlab function part2_sim5/Observer/Extended Kalman Filter/Extended Kalman Filter ==
  data: P_hat output; y input; tau input; EKFData parameter; x_hat output; P_bar output; x_bar output; P_bar input; x_bar input
function [P_hat, x_hat, P_bar, x_bar] = ExtendedKalmanFilter(y, tau,EKFData,...
    P_bar, x_bar)

persistent Aw B_kf H_kf E_kf M_inv D...
     R_kf Q_kf... 
    h_step Tb Phi 

   [Aw,B_kf,H_kf,E_kf,R_kf,Q_kf, M_inv, D, ~, ~, h_step, Tb] = ...
        deal(EKFData.Aw, EKFData.B_kf, EKFData.H_kf, EKFData.E_kf,...
        EKFData.R_kf,EKFData.Q_kf,EKFData.M_inv,EKFData.D,EKFData.Zetan,...
        EKFData.Wn, EKFData.h_step, EKFData.Tb);

% if isempty(init_flag)
%     init_flag = 1;
%     P_bar = EKFData.P0;
%     x_bar= EKFData.x0;
% end

%Computing kalman gain based on prediction
K = (P_bar*H_kf')/((H_kf*P_bar*H_kf' + R_kf));

%Update the error covariance matrix with prediction estimate
P_hat = (eye(15) - K*H_kf)*P_bar*(eye(15)-K*H_kf)' + K*R_kf*K';

%Correction: Update predicted estimate with measurement
x_hat = x_bar + K*(y-H_kf*x_bar);

%Linearization
Phi = eye(15) + h_step*Jacobi(x_hat, Aw, Tb,M_inv,D);
gamma = h_step*E_kf;

%Prediction
P_bar = Phi*P_hat*Phi' + gamma*Q_kf*gamma';
x_bar = x_hat + h_step*(f(x_hat,Aw,Tb,M_inv,D) + B_kf*tau);

% x =[xi_1 til x_6, N(7), E(8), psi(9),b1(10), b2(11), b3(12), u(13),
% v(14),r(15)], n=15 states
end

%% Jacobi
function [J] = Jacobi(x_hat, Aw, Tb, M_inv, D)
J = [Aw zeros(6,9);zeros(9,15)];
% J(1,:) = [0 0 0 1 0 0    0 0 0      0 0 0       0 0 0];
% J(2,:) = [0 0 0 0 1 0    0 0 0      0 0 0       0 0 0];
% J(3,:) = [0 0 0 0 0 1    0 0 0      0 0 0       0 0 0];
% J(4,:) = [-(Wn(1))^2-2*Zetan(1)*Wn(1) 0 0      0 0 0   0 0 0   0 0 0   0 0 0];
% J(5,:) = [0 -(Wn(2))^2-2*Zetan(2)*Wn(2) 0      0 0 0   0 0 0   0 0 0   0 0 0];
% J(6,:) = [0 0 -(Wn(3))^2-2*Zetan(3)*Wn(3)      0 0 0   0 0 0   0 0 0   0 0 0];

J(7,:) = [0 0 0 0 0 0   0 0 -sin(x_hat(9))*x_hat(13)-cos(x_hat(9))*x_hat(14)     0 0 0   cos(x_hat(9)) -sin(x_hat(9)) 0]; 
J(8,:) = [0 0 0 0 0 0   0 0 cos(x_hat(9))*x_hat(13)-sin(x_hat(9))*x_hat(14)      0 0 0   sin(x_hat(9)) cos(x_hat(9))  0];
J(9,:) = [0 0 0 0 0 0   0 0 0                           0 0 0   0 0 1];

J(10,:) = [0 0 0 0 0 0  0 0 0   inv(-Tb(1)) 0 0    0 0 0];
J(11,:) = [0 0 0 0 0 0  0 0 0   0 inv(-Tb(2)) 0    0 0 0];
J(12,:) = [0 0 0 0 0 0  0 0 0   0 0 inv(-Tb(3))    0 0 0];

J(13,:) = [0 0 0 0 0 0  0 0 M_inv(1,1)*(-sin(x_hat(9))*x_hat(10)+cos(x_hat(9))*x_hat(11))   M_inv(1,1)*cos(x_hat(9)) M_inv(1,1)*sin(x_hat(9)) 0               -M_inv(1,1)*D(1,1) 0 0];
J(14,:) = [0 0 0 0 0 0  0 0 M_inv(2,2)*(-cos(x_hat(9))*x_hat(10)-sin(x_hat(9))*x_hat(11))   M_inv(2,2)*sin(x_hat(9)) M_inv(2,2)*cos(x_hat(9)) M_inv(2,3)      0 -M_inv(2,2)*D(2,2) -M_inv(2,3)*D(3,3)];
J(15,:) = [0 0 0 0 0 0  0 0 M_inv(3,2)*(-cos(x_hat(9))*x_hat(10)-cos(x_hat(9))*x_hat(11))   M_inv(3,2)*(-sin(x_hat(9))) M_inv(3,2)*cos(x_hat(9)) M_inv(3,3)    0 M_inv(3,2) M_inv(3,3)*D(3,3)];
 end
                          

function f = f(x_hat, Aw, Tb, M_inv, D)
    Tb_inv = (Tb).^(-1);

    f = zeros(15,1);
    f(1:6,1) = Aw*x_hat(1:6,1);
    f(7:9,1) = R(x_hat(9,1))*x_hat(13:15,1);
    f(10:12,1) = -(Tb_inv)*x_hat(10:12,1);
    f(13:15,1) = (-M_inv*D*x_hat(13:15,1))...
    + M_inv*(R(x_hat(9,1)))'*x_hat(10:12,1);
end

function Rotation = R(psi)
     Rotation = [cos(psi) -sin(psi) 0;
            sin(psi) cos(psi) 0;
            0   0   1];
end
